simulink model "rzs10thnew2021b"  (R2021b)
settings: Solver=FixedStepDiscrete  StartTime=0.0  StopTime=10.0  FixedStep=0.001  RelTol=1e-3  EnableMultiTasking=on
values from neighbouring files (symbols this model uses):
  F = 0.0    [rzdatabase.sldd]
  T = 1.0    [rzdatabase.sldd]
libraries: simulink x143, hdlsllib x95, spsEdgeDetectorLib x3
(part 2 of 3)

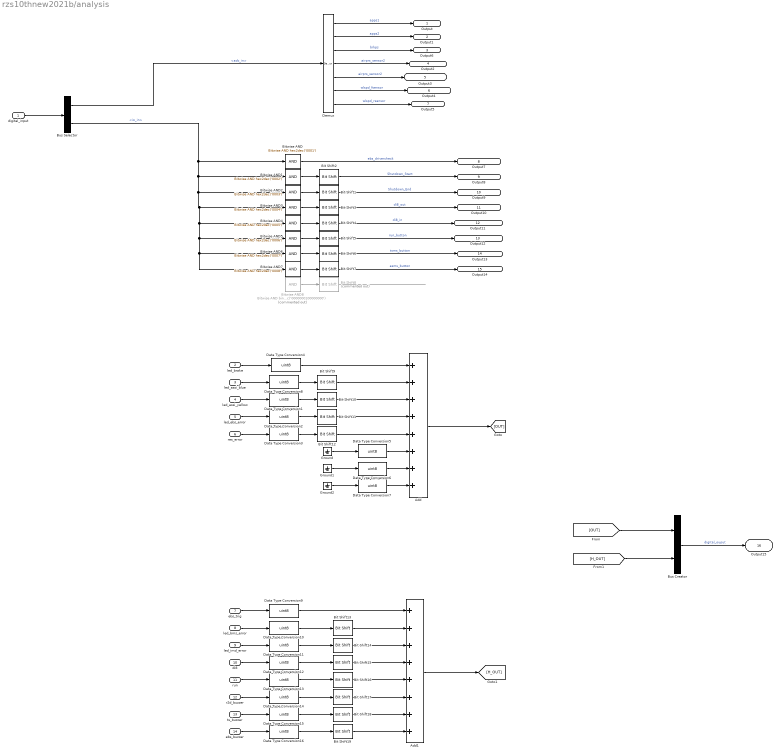
== system rzs10thnew2021b/analysis ==
  digital_input : Inport
  led_brake : Inport  Port=2
  led_assi_blue : Inport  Port=3
  led_assi_yellow : Inport  Port=4
  led_ebs_error : Inport  Port=5
  res_error : Inport  Port=6
  ebs_trig : Inport  Port=7
  led_bms_error : Inport  Port=8
  led_imd_error : Inport  Port=9
  di8 : Inport  Port=10
  run : Inport  Port=11
  r2d_buzzer : Inport  Port=12
  ts_buzzer : Inport  Port=13
  ebs_buzzer : Inport  Port=14
  Add : Sum  Inputs=++++++++
  Add1 : Sum  Inputs=++++++++
  Bit Shift1 : hdlsllib/Logic and Bit Operations/Bit Shift  mode=Shift Right Logical  N=2
  Bit Shift10 : hdlsllib/Logic and Bit Operations/Bit Shift  mode=Shift Right Logical  N=2
  Bit Shift11 : hdlsllib/Logic and Bit Operations/Bit Shift  mode=Shift Right Logical  N=3
  Bit Shift12 : hdlsllib/Logic and Bit Operations/Bit Shift  mode=Shift Right Logical  N=4
  Bit Shift13 : hdlsllib/Logic and Bit Operations/Bit Shift  mode=Shift Left Logical  N=1
  Bit Shift14 : hdlsllib/Logic and Bit Operations/Bit Shift  mode=Shift Left Logical  N=2
  Bit Shift15 : hdlsllib/Logic and Bit Operations/Bit Shift  mode=Shift Left Logical  N=3
  Bit Shift16 : hdlsllib/Logic and Bit Operations/Bit Shift  mode=Shift Left Logical  N=4
  Bit Shift17 : hdlsllib/Logic and Bit Operations/Bit Shift  mode=Shift Left Logical  N=5
  Bit Shift18 : hdlsllib/Logic and Bit Operations/Bit Shift  mode=Shift Left Logical  N=6
  Bit Shift19 : hdlsllib/Logic and Bit Operations/Bit Shift  mode=Shift Left Logical  N=7
  Bit Shift2 : hdlsllib/Logic and Bit Operations/Bit Shift  mode=Shift Right Logical  N=1
  Bit Shift3 : hdlsllib/Logic and Bit Operations/Bit Shift  mode=Shift Right Logical  N=3
  Bit Shift4 : hdlsllib/Logic and Bit Operations/Bit Shift  mode=Shift Right Logical  N=4
  Bit Shift5 : hdlsllib/Logic and Bit Operations/Bit Shift  mode=Shift Right Logical  N=5
  Bit Shift6 : hdlsllib/Logic and Bit Operations/Bit Shift  mode=Shift Right Logical  N=6
  Bit Shift7 : hdlsllib/Logic and Bit Operations/Bit Shift  mode=Shift Right Logical  N=7
  Bit Shift8 : hdlsllib/Logic and Bit Operations/Bit Shift  Commented=on  mode=Shift Right Logical  N=8
  Bit Shift9 : hdlsllib/Logic and Bit Operations/Bit Shift  mode=Shift Left Logical  N=1
  Bitwise AND : simulink/Logic and Bit Operations/Bitwise Operator  logicop=AND  UseBitMask=on  BitMask=hex2dec('0001')  BitMaskRealWorld=Stored Integer
  Bitwise AND1 : simulink/Logic and Bit Operations/Bitwise Operator  logicop=AND  UseBitMask=on  BitMask=hex2dec('0002')  BitMaskRealWorld=Stored Integer
  Bitwise AND2 : simulink/Logic and Bit Operations/Bitwise Operator  logicop=AND  UseBitMask=on  BitMask=hex2dec('0003')  BitMaskRealWorld=Stored Integer
  Bitwise AND3 : simulink/Logic and Bit Operations/Bitwise Operator  logicop=AND  UseBitMask=on  BitMask=hex2dec('0004')  BitMaskRealWorld=Stored Integer
  Bitwise AND4 : simulink/Logic and Bit Operations/Bitwise Operator  logicop=AND  UseBitMask=on  BitMask=hex2dec('0005')  BitMaskRealWorld=Stored Integer
  Bitwise AND5 : simulink/Logic and Bit Operations/Bitwise Operator  logicop=AND  UseBitMask=on  BitMask=hex2dec('0006')  BitMaskRealWorld=Stored Integer
  Bitwise AND6 : simulink/Logic and Bit Operations/Bitwise Operator  logicop=AND  UseBitMask=on  BitMask=hex2dec('0007')  BitMaskRealWorld=Stored Integer
  Bitwise AND7 : simulink/Logic and Bit Operations/Bitwise Operator  logicop=AND  UseBitMask=on  BitMask=hex2dec('0008')  BitMaskRealWorld=Stored Integer
  Bitwise AND8 : simulink/Logic and Bit Operations/Bitwise Operator  Commented=on  logicop=AND  UseBitMask=on  BitMask=bin2dec('0000000100000000')  BitMaskRealWorld=Stored Integer
  Bus Creator : BusCreator  Inputs=2  OutDataTypeStr=Bus: VCU_OUT_PAR  NonVirtualBus=on
      settings: InheritFromInputs=off
  Bus Selector : BusSelector  OutputSignals=adc_in,io_in
  Data Type Conversion{1..16} (16 alike) : DataTypeConversion  OutDataTypeStr=uint8
  Demux : Demux  Outputs=7
  Ground : Ground
  Ground1 : Ground
  Ground2 : Ground
  Output : Outport
  Output1 : Outport  Port=2
  Output6 : Outport  Port=3
  Output2 : Outport  Port=4
  Output3 : Outport  Port=5
  Output4 : Outport  Port=6
  Output5 : Outport  Port=7
  Output7 : Outport  Port=8
  Output8 : Outport  Port=9
  Output9 : Outport  Port=10
  Output10 : Outport  Port=11
  Output11 : Outport  Port=12
  Output12 : Outport  Port=13
  Output13 : Outport  Port=14
  Output14 : Outport  Port=15
  Output15 : Outport  Port=16
  wires:
  Bitwise AND1/1 -> Bit Shift2/1
  Bitwise AND2/1 -> Bit Shift1/1
  Bitwise AND3/1 -> Bit Shift3/1
  Bitwise AND4/1 -> Bit Shift4/1
  Bitwise AND5/1 -> Bit Shift5/1
  Bitwise AND6/1 -> Bit Shift6/1
  Bitwise AND7/1 -> Bit Shift7/1
  Bitwise AND8/1 -> Bit Shift8/1
  Bit Shift2/1 -> Output8/1  "Shutdown_Start"
  Bit Shift1/1 -> Output9/1  "Shutdown_End"
  Bit Shift3/1 -> Output10/1  "di8_out"
  Bit Shift4/1 -> Output11/1  "di8_in"
  Bit Shift5/1 -> Output12/1  "run_button"
  Bit Shift6/1 -> Output13/1  "tsms_button"
  Bit Shift7/1 -> Output14/1  "asms_button"
  Bit Shift8/1 -> ?
  Bitwise AND/1 -> Output7/1  "ebs_drivercheck"
  Ground2/1 -> Data Type Conversion7/1
  Ground1/1 -> Data Type Conversion6/1
  Ground/1 -> Data Type Conversion5/1
  Bit Shift13/1 -> Add1/2
  Bit Shift14/1 -> Add1/3
  Bit Shift15/1 -> Add1/4
  Bit Shift16/1 -> Add1/5
  Bit Shift17/1 -> Add1/6
  Bit Shift18/1 -> Add1/7
  Bit Shift19/1 -> Add1/8
  led_brake/1 -> Data Type Conversion4/1
  Data Type Conversion4/1 -> Add/1
  Bit Shift9/1 -> Add/2
  Bit Shift10/1 -> Add/3
  Bit Shift11/1 -> Add/4
  Bit Shift12/1 -> Add/5
  Data Type Conversion5/1 -> Add/6
  Data Type Conversion6/1 -> Add/7
  Data Type Conversion7/1 -> Add/8
  led_assi_blue/1 -> Data Type Conversion8/1
  Data Type Conversion8/1 -> Bit Shift9/1
  led_assi_yellow/1 -> Data Type Conversion1/1
  Data Type Conversion1/1 -> Bit Shift10/1
  led_ebs_error/1 -> Data Type Conversion2/1
  Data Type Conversion2/1 -> Bit Shift11/1
  res_error/1 -> Data Type Conversion3/1
  Data Type Conversion3/1 -> Bit Shift12/1
  ebs_trig/1 -> Data Type Conversion9/1
  Data Type Conversion9/1 -> Add1/1
  led_bms_error/1 -> Data Type Conversion10/1
  Data Type Conversion10/1 -> Bit Shift13/1
  led_imd_error/1 -> Data Type Conversion11/1
  Data Type Conversion11/1 -> Bit Shift14/1
  di8/1 -> Data Type Conversion12/1
  Data Type Conversion12/1 -> Bit Shift15/1
  run/1 -> Data Type Conversion13/1
  Data Type Conversion13/1 -> Bit Shift16/1
  r2d_buzzer/1 -> Data Type Conversion14/1
  Data Type Conversion14/1 -> Bit Shift17/1
  ts_buzzer/1 -> Data Type Conversion15/1
  Data Type Conversion15/1 -> Bit Shift18/1
  ebs_buzzer/1 -> Data Type Conversion16/1
  Data Type Conversion16/1 -> Bit Shift19/1
  Demux/1 -> Output/1  "apps1"
  Demux/2 -> Output1/1  "apps2"
  Demux/3 -> Output6/1  "brkps"
  Demux/5 -> Output3/1  "airprs_sensor2"
  Demux/6 -> Output4/1  "wlspd_fsensor"
  Demux/7 -> Output5/1  "wlspd_rsensor"
  Bus Creator/1 -> Output15/1  "digital_ouput"
  Demux/4 -> Output2/1  "airprs_sensor2"
  Add1/1 -> [H_OUT]
  Add/1 -> [OUT]
  [H_OUT] -> Bus Creator/2
  [OUT] -> Bus Creator/1
  Bus Selector/1 -> Demux/1  "<adc_in>"
  Bus Selector/2 -> Bitwise AND7/1, Bitwise AND6/1, Bitwise AND5/1, Bitwise AND4/1, Bitwise AND3/1, Bitwise AND2/1, Bitwise AND1/1, Bitwise AND/1  "<io_in>"
  digital_input/1 -> Bus Selector/1

== system rzs10thnew2021b/AMI_CAN/AMI_Receivemsg ==
  AMI_Tx : Inport
  Bit Shift : hdlsllib/Logic and Bit Operations/Bit Shift  mode=Shift Right Logical  N=4
  Bitwise AND : simulink/Logic and Bit Operations/Bitwise Operator  logicop=AND  UseBitMask=on  BitMask=bin2dec('11110000')  BitMaskRealWorld=Stored Integer
  Demux : Demux  Outputs=8
  Mux : Mux  Inputs=8
  ami_astask : Outport
  Output : Outport  Port=2
  wires:
  Demux/6 -> Mux/6
  Demux/2 -> Mux/2
  Demux/4 -> Mux/4
  AMI_Tx/1 -> Demux/1
  Demux/7 -> Mux/7
  Demux/5 -> Mux/5
  Demux/8 -> Mux/8
  Demux/3 -> Mux/3
  Demux/1 -> Mux/1, Bitwise AND/1
  Bitwise AND/1 -> Bit Shift/1
  Bit Shift/1 -> ami_astask/1
  Mux/1 -> Output/1

== system rzs10thnew2021b/AMI_CAN/AMI_Transmitmsg ==
  as_flag_state : Inport
  task_finish : Inport  Port=2
  Add1 : Sum
  Bit Shift : hdlsllib/Logic and Bit Operations/Bit Shift  mode=Shift Left Logical  N=1
  Bitwise AND : simulink/Logic and Bit Operations/Bitwise Operator  logicop=AND  UseBitMask=on  BitMask=bin2dec('01111111')  BitMaskRealWorld=Stored Integer
  Bus Selector : BusSelector  OutputSignals=as_off_flag,manual_driving_flag,as_ready_flag,r2d_flag,as_driving_flag,as_finished_flag,as_emergency_flag
  Chart : Stateflow chart  TreatAsAtomicUnit=on
  Ground{,1..6} (7 alike) : Ground
  Mux : Mux  Inputs=8
  Signal Conversion : SignalConversion  OverrideOpt=off
  Output : Outport
  wires:
  as_flag_state/1 -> Bus Selector/1
  Bitwise AND/1 -> Bit Shift/1
  Bit Shift/1 -> Add1/1
  task_finish/1 -> Add1/2
  Add1/1 -> Mux/1
  Bus Selector/1 -> Chart/1(as_off_flag)  "<as_off_flag>"
  Bus Selector/2 -> Chart/2(munual_driving_flag)  "<manual_driving_flag>"
  Bus Selector/3 -> Chart/3(as_ready_flag)  "<as_ready_flag>"
  Bus Selector/4 -> Chart/4(r2d_flag)  "<r2d_flag>"
  Bus Selector/5 -> Chart/5(as_driving_flag)  "<as_driving_flag>"
  Bus Selector/6 -> Chart/6(as_finished_flag)  "<as_finished_flag>"
  Bus Selector/7 -> Chart/7(as_emergency_flag)  "<as_emergency_flag>"
  Chart/1(ami_process) -> Bitwise AND/1
  Ground/1 -> Mux/2
  Ground1/1 -> Mux/3
  Ground2/1 -> Mux/4
  Ground3/1 -> Mux/5
  Ground4/1 -> Mux/6
  Ground5/1 -> Mux/7
  Ground6/1 -> Mux/8
  Mux/1 -> Signal Conversion/1
  Signal Conversion/1 -> Output/1

== system rzs10thnew2021b/ASB_Selfcheck/Brake_Sensor_Check ==
  note: 下四路为有效制动阈值油压
  note: 上四路油压信号阈值为非制动状态油压
  note: 所有常数待定
  airprs_sensor1 : Inport
  oilprs_frsensor : Inport  Port=2
  oilprs_rrsensor : Inport  Port=3
  oilprs_flsensor : Inport  Port=4
  oilprs_rlsensor : Inport  Port=5
  Compare To Constant : simulink/Logic and Bit Operations/Compare To Constant  relop=>=  const=0.74  OutDataTypeStr=boolean
  Compare To Constant{1,3,5,7} (4 alike) : simulink/Logic and Bit Operations/Compare To Constant  relop=>=  const=0.848  OutDataTypeStr=boolean
  Compare To Constant{2,4,6,8} (4 alike) : simulink/Logic and Bit Operations/Compare To Constant  relop=>=  const=0.742  OutDataTypeStr=boolean
  Logical Operator : Logic  Inputs=5  AllPortsSameDT=off  OutDataTypeStr=boolean
  Logical Operator1 : Logic  Inputs=4  AllPortsSameDT=off  OutDataTypeStr=boolean
  brksensor_check : Outport
  brake_on : Outport  Port=2
  wires:
  airprs_sensor1/1 -> Compare To Constant/1
  oilprs_frsensor/1 -> Compare To Constant5/1, Compare To Constant1/1
  oilprs_rrsensor/1 -> Compare To Constant7/1, Compare To Constant3/1
  oilprs_flsensor/1 -> Compare To Constant6/1, Compare To Constant2/1
  oilprs_rlsensor/1 -> Compare To Constant8/1, Compare To Constant4/1
  Compare To Constant3/1 -> Logical Operator/3
  Compare To Constant/1 -> Logical Operator/1
  Compare To Constant1/1 -> Logical Operator/2
  Compare To Constant2/1 -> Logical Operator/4
  Compare To Constant4/1 -> Logical Operator/5
  Logical Operator/1 -> brksensor_check/1
  Logical Operator1/1 -> brake_on/1
  Compare To Constant5/1 -> Logical Operator1/1
  Compare To Constant7/1 -> Logical Operator1/2
  Compare To Constant6/1 -> Logical Operator1/3
  Compare To Constant8/1 -> Logical Operator1/4

== system rzs10thnew2021b/ASB_Selfcheck/EBS_On_Check ==
  airprs_sensor2 : Inport
  Compare To Constant : simulink/Logic and Bit Operations/Compare To Constant  relop=>=  const=0.9  OutDataTypeStr=boolean
  ebs_working : Outport
  wires:
  airprs_sensor2/1 -> Compare To Constant/1
  Compare To Constant/1 -> ebs_working/1

== system rzs10thnew2021b/AS_Stateflow/Car_Spdzero_Check ==
  wlspd_fsensor : Inport
  wlspd_hsensor : Inport  Port=2
  Compare To Constant : simulink/Logic and Bit Operations/Compare To Constant  relop===  const=0  OutDataTypeStr=boolean
  Compare To Constant1 : simulink/Logic and Bit Operations/Compare To Constant  relop===  const=0  OutDataTypeStr=boolean
  Dead Zone : DeadZone  SaturateOnIntegerOverflow=on
  Dead Zone1 : DeadZone  SaturateOnIntegerOverflow=on
  Logical Operator : Logic  AllPortsSameDT=off  OutDataTypeStr=boolean
  car_spdzero : Outport
  wires:
  wlspd_fsensor/1 -> Dead Zone/1
  wlspd_hsensor/1 -> Dead Zone1/1
  Dead Zone/1 -> Compare To Constant/1
  Dead Zone1/1 -> Compare To Constant1/1
  Compare To Constant/1 -> Logical Operator/1
  Compare To Constant1/1 -> Logical Operator/2
  Logical Operator/1 -> car_spdzero/1

== system rzs10thnew2021b/EPS/EPS_ReceiveMsg ==
  canb_epssendmsg1 : Inport
  canb_epssendmsg2 : Inport  Port=2
  EPS_Send_Msg1 : Subsystem
  EPS_Send_Msg2 : Subsystem
  canb_epssendmsg1signal : Outport
  canb_epssendmsg2signal : Outport  Port=2
  wires:
  canb_epssendmsg1/1 -> EPS_Send_Msg1/1(canb_epssendmsg1)
  EPS_Send_Msg1/1(canb_epssendmsg1signal) -> canb_epssendmsg1signal/1
  canb_epssendmsg2/1 -> EPS_Send_Msg2/1(canb_epssendmsg2)
  EPS_Send_Msg2/1(canb_epssendmsg2signal) -> canb_epssendmsg2signal/1

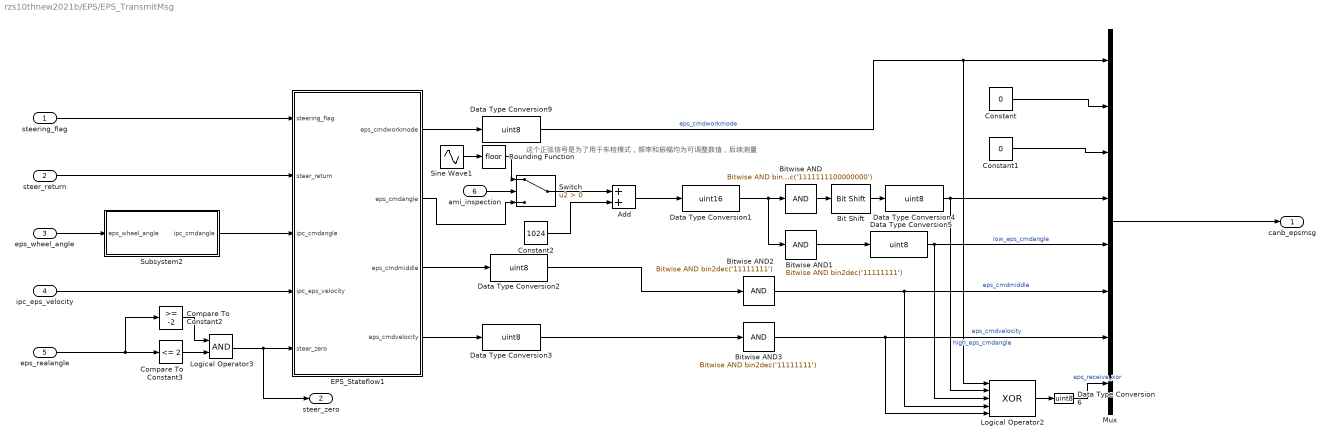
== system rzs10thnew2021b/EPS/EPS_TransmitMsg ==
  note: 这个正弦信号是为了用于车检模式，频率和振幅均为可调整数值，后续测量
  steering_flag : Inport
  steer_return : Inport  Port=2
  eps_wheel_angle : Inport  Port=3
  ipc_eps_velocity : Inport  Port=4
  eps_realangle : Inport  Port=5
  ami_inspection : Inport  Port=6
  Add : Sum
  Bit Shift : hdlsllib/Logic and Bit Operations/Bit Shift  mode=Shift Right Logical  N=8
  Bitwise AND : simulink/Logic and Bit Operations/Bitwise Operator  logicop=AND  UseBitMask=on  BitMask=bin2dec('1111111100000000')  BitMaskRealWorld=Stored Integer
  Bitwise AND1 : simulink/Logic and Bit Operations/Bitwise Operator  logicop=AND  UseBitMask=on  BitMask=bin2dec('11111111')  BitMaskRealWorld=Stored Integer
  Bitwise AND2 : simulink/Logic and Bit Operations/Bitwise Operator  logicop=AND  UseBitMask=on  BitMask=bin2dec('11111111')  BitMaskRealWorld=Stored Integer
  Bitwise AND3 : simulink/Logic and Bit Operations/Bitwise Operator  logicop=AND  UseBitMask=on  BitMask=bin2dec('11111111')  BitMaskRealWorld=Stored Integer
  Compare To Constant2 : simulink/Logic and Bit Operations/Compare To Constant  relop=>=  const=-2  OutDataTypeStr=boolean
  Compare To Constant3 : simulink/Logic and Bit Operations/Compare To Constant  relop=<=  const=2  OutDataTypeStr=boolean
  Constant : Constant  Value=0  OutDataTypeStr=uint8
  Constant1 : Constant  Value=0  OutDataTypeStr=uint8
  Constant2 : Constant  Value=1024  OutDataTypeStr=double
  Data Type Conversion1 : DataTypeConversion  OutDataTypeStr=uint16
  Data Type Conversion{2..6,9} (6 alike) : DataTypeConversion  OutDataTypeStr=uint8
  EPS_Stateflow1 : Stateflow chart  TreatAsAtomicUnit=on
  Logical Operator2 : Logic  Operator=XOR  Inputs=5  AllPortsSameDT=off  OutDataTypeStr=boolean
  Logical Operator3 : Logic  AllPortsSameDT=off  OutDataTypeStr=boolean
  Mux : Mux  Inputs=8
  Rounding Function : Rounding
  Sine Wave1 : Sin  Amplitude=90
  Subsystem2 : Subsystem
  Switch : Switch  Criteria=u2 > Threshold
  canb_epsmsg : Outport
  steer_zero : Outport  Port=2
  wires:
  Data Type Conversion5/1 -> Logical Operator2/3, Mux/5  "low_eps_cmdangle"
  Data Type Conversion9/1 -> Logical Operator2/1, Mux/1  "eps_cmdworkmode"
  Bitwise AND3/1 -> Logical Operator2/5, Mux/7  "eps_cmdvelocity"
  Compare To Constant3/1 -> Logical Operator3/2
  Data Type Conversion3/1 -> Bitwise AND3/1
  Bit Shift/1 -> Data Type Conversion4/1
  eps_realangle/1 -> Compare To Constant2/1, Compare To Constant3/1
  Data Type Conversion1/1 -> Bitwise AND/1, Bitwise AND1/1
  EPS_Stateflow1/4(eps_cmdvelocity) -> Data Type Conversion3/1
  Logical Operator3/1 -> steer_zero/1, EPS_Stateflow1/5(steer_zero)
  Bitwise AND2/1 -> Logical Operator2/4, Mux/6  "eps_cmdmiddle"
  EPS_Stateflow1/3(eps_cmdmiddle) -> Data Type Conversion2/1
  Constant1/1 -> Mux/3
  Bitwise AND/1 -> Bit Shift/1
  Data Type Conversion4/1 -> Mux/4, Logical Operator2/2  "high_eps_cmdangle"
  eps_wheel_angle/1 -> Subsystem2/1(eps_wheel_angle)
  Data Type Conversion2/1 -> Bitwise AND2/1
  Compare To Constant2/1 -> Logical Operator3/1
  Logical Operator2/1 -> Data Type Conversion6/1
  steer_return/1 -> EPS_Stateflow1/2(steer_return)
  EPS_Stateflow1/1(eps_cmdworkmode) -> Data Type Conversion9/1
  Bitwise AND1/1 -> Data Type Conversion5/1
  ipc_eps_velocity/1 -> EPS_Stateflow1/4(ipc_eps_velocity)
  Constant/1 -> Mux/2
  Subsystem2/1(ipc_cmdangle) -> EPS_Stateflow1/3(ipc_cmdangle)
  Mux/1 -> canb_epsmsg/1
  steering_flag/1 -> EPS_Stateflow1/1(steering_flag)
  Add/1 -> Data Type Conversion1/1
  Constant2/1 -> Add/2
  Data Type Conversion6/1 -> Mux/8  "eps_receive_xor"
  ami_inspection/1 -> Switch/2
  Switch/1 -> Add/1
  EPS_Stateflow1/2(eps_cmdangle) -> Switch/3
  Rounding Function/1 -> Switch/1
  Sine Wave1/1 -> Rounding Function/1

== system rzs10thnew2021b/ESP/ESP_ReceiveMsg ==
  canb_esp_t01 : Inport
  canb_esp_t03 : Inport  Port=2
  canb_esp_t06 : Inport  Port=3
  canb_esp_t07 : Inport  Port=4
  Bus Selector : BusSelector  OutputSignals=lifeSig
  ESP_T_01 : Subsystem
  ESP_T_03 : Subsystem
  ESP_T_06 : Subsystem
  ESP_T_07 : Subsystem
  Subsystem : Subsystem
  ESP_T_01sigal : Outport
  ESP_T_03signal : Outport  Port=2
  ESP_T_06signal : Outport  Port=3
  ESP_T_07signal : Outport  Port=4
  brkmotor_check : Outport  Port=5
  wires:
  canb_esp_t01/1 -> ESP_T_01/1(canb_esp_t01)
  ESP_T_01/1(ESP_T_01sigal) -> ESP_T_01sigal/1
  canb_esp_t03/1 -> ESP_T_03/1(canb_esp_t03)
  canb_esp_t06/1 -> ESP_T_06/1(canb_esp_t06)
  ESP_T_06/1(ESP_T_06signal) -> ESP_T_06signal/1
  canb_esp_t07/1 -> ESP_T_07/1(canb_esp_t07)
  ESP_T_07/1(ESP_T_07signal) -> ESP_T_07signal/1
  Subsystem/1(brkmotor_check) -> brkmotor_check/1
  ESP_T_03/1(ESP_T_03signal) -> Bus Selector/1, ESP_T_03signal/1
  Bus Selector/1 -> Subsystem/1(lifesig)  "<lifeSig>"

== system rzs10thnew2021b/ESP/ESP_TransmitMsg ==
  ipc_esp_pressure : Inport
  brake_flag : Inport  Port=2
  lifeSig : Inport  Port=3
  checkSum : Inport  Port=4
  ESP_R_00 : Subsystem
  canb_esp_r00 : Outport
  wires:
  ipc_esp_pressure/1 -> ESP_R_00/1(ipc_esp_pressure)
  brake_flag/1 -> ESP_R_00/2(brake_flag)
  ESP_R_00/1(canb_esp_r00) -> canb_esp_r00/1
  checkSum/1 -> ESP_R_00/4(checkSum)
  lifeSig/1 -> ESP_R_00/3(lifeSig)

== system rzs10thnew2021b/IPC/IPC_ReceiveMsg ==
  ipc_resgo : Inport
  ipc_resstop : Inport  Port=2
  ipc_astask : Inport  Port=3
  IPC_Rx_Msg : Subsystem
  canb_ipcrxmsg : Outport
  wires:
  ipc_resgo/1 -> IPC_Rx_Msg/1(ipc_resgo)
  ipc_resstop/1 -> IPC_Rx_Msg/2(ipc_resstop)
  ipc_astask/1 -> IPC_Rx_Msg/3(ipc_astask)
  IPC_Rx_Msg/1(canb_ipcrxmsg) -> canb_ipcrxmsg/1

== system rzs10thnew2021b/IPC/IPC_TransmitMsg ==
  canb_ipctsmsg1 : Inport
  canb_ipctsmsg2 : Inport  Port=2
  IPC_Tx_Msg1 : Subsystem
  IPC_Tx_Msg2 : Subsystem
  ipc_esp_pressure : Outport
  ipc_motor_torque : Outport  Port=2
  ipc_eps_angle : Outport  Port=3
  ipc_eps_velocity : Outport  Port=4
  ipc_err : Outport  Port=5
  task_finish : Outport  Port=6
  wires:
  canb_ipctsmsg1/1 -> IPC_Tx_Msg1/1(canb_ipctsmsg1)
  IPC_Tx_Msg1/1(ipc_esp_pressure) -> ipc_esp_pressure/1
  IPC_Tx_Msg1/2(ipc_motor_torque) -> ipc_motor_torque/1
  canb_ipctsmsg2/1 -> IPC_Tx_Msg2/1(canb_ipctsmsg2)
  IPC_Tx_Msg2/2(ipc_eps_velocity) -> ipc_eps_velocity/1
  IPC_Tx_Msg2/1(ipc_eps_angle) -> ipc_eps_angle/1
  IPC_Tx_Msg2/3(ipc_err) -> ipc_err/1
  IPC_Tx_Msg2/4(task_finish) -> task_finish/1

== system rzs10thnew2021b/LED_Control/BMS_LED ==
  bms_error : Inport
  imd_error : Inport  Port=2
  BMS_LED : Stateflow chart  TreatAsAtomicUnit=on
  IMD_LED : Stateflow chart  TreatAsAtomicUnit=on
  led_bms_error : Outport
  led_imd_error : Outport  Port=2
  wires:
  bms_error/1 -> BMS_LED/1(bms_error)
  imd_error/1 -> IMD_LED/1(imd_error)
  BMS_LED/1(led_bms_error) -> led_bms_error/1  "led_bms_error"
  IMD_LED/1(led_imd_error) -> led_imd_error/1  "led_imd_error"

== system rzs10thnew2021b/LED_Control/EBS_LED ==
  note: 液压元件失效
  note: 手动阀未关
  note: 前气路故障
  note: 上电亮灯
  note: 气动元件检测与气压检测
  note: 油压检测
  res_stop : Inport
  res_communication : Inport  Port=2
  Shutdown_Start : Inport  Port=3
  Shutdown_End : Inport  Port=4
  sensor_signal : Inport  Port=5
  ESP_T_03signal : Inport  Port=6
  asms_button : Inport  Port=7
  Bus Selector : BusSelector  OutputSignals=airprs_sensor1,airprs_sensor2
  Bus Selector1 : BusSelector  OutputSignals=oilprs_flsensor,oilprs_frsensor,oilprs_rlsensor,oilprs_rrsensor
  Compare To Constant{,3..6} (5 alike) : simulink/Logic and Bit Operations/Compare To Constant  relop=<=  const=0.11  OutDataTypeStr=boolean
  Compare To Constant1 : simulink/Logic and Bit Operations/Compare To Constant  relop=<=  const=0.5  OutDataTypeStr=boolean
  Compare To Constant2 : simulink/Logic and Bit Operations/Compare To Constant  relop=>=  const=0.78  OutDataTypeStr=boolean
  Enabled Subsystem : Subsystem  TreatAsAtomicUnit=on
  Logical Operator : Logic  Operator=OR  Inputs=5  AllPortsSameDT=off  OutDataTypeStr=boolean
  Logical Operator2 : Logic  Inputs=4  AllPortsSameDT=off  OutDataTypeStr=boolean
  Logical Operator3 : Logic  Operator=OR  Inputs=4  AllPortsSameDT=off  OutDataTypeStr=boolean
  Shutdown_Button : Stateflow chart  TreatAsAtomicUnit=on
  display : Stateflow chart  TreatAsAtomicUnit=on
  led_ebs_error : Outport
  wires:
  Compare To Constant5/1 -> Logical Operator3/3
  Bus Selector/2 -> Compare To Constant1/1, Compare To Constant2/1  "<airprs_sensor2>"
  Compare To Constant2/1 -> Enabled Subsystem/1(In1)
  Compare To Constant1/1 -> Logical Operator/2
  Logical Operator/1 -> led_ebs_error/1
  Bus Selector1/4 -> Compare To Constant6/1  "<oilprs_rrsensor>"
  Compare To Constant4/1 -> Logical Operator3/2
  Bus Selector/1 -> Compare To Constant/1  "<airprs_sensor1>"
  Compare To Constant6/1 -> Logical Operator3/4
  Bus Selector1/1 -> Compare To Constant3/1  "<oilprs_flsensor>"
  display/1(spark) -> Logical Operator/5
  Logical Operator3/1 -> Logical Operator/4
  asms_button/1 -> Logical Operator2/4
  Logical Operator2/1 -> Enabled Subsystem/Enable
  Compare To Constant/1 -> Logical Operator/1
  Enabled Subsystem/1(Out1) -> Logical Operator/3
  Shutdown_Button/1(shutdown_flag) -> Logical Operator2/3
  Compare To Constant3/1 -> Logical Operator3/1
  Bus Selector1/2 -> Compare To Constant4/1  "<oilprs_frsensor>"
  Bus Selector1/3 -> Compare To Constant5/1  "<oilprs_rlsensor>"
  ESP_T_03signal/1 -> Bus Selector1/1
  res_stop/1 -> Logical Operator2/1
  res_communication/1 -> Logical Operator2/2
  Shutdown_End/1 -> Shutdown_Button/2(Shutdown_End)
  Shutdown_Start/1 -> Shutdown_Button/1(Shutdown_Start)
  sensor_signal/1 -> Bus Selector/1

== system rzs10thnew2021b/LED_Control/Subsystem ==
  as_led_blue1 : Inport
  asms_button : Inport  Port=2
  Constant : Constant  Value=0
  Constant1 : Constant  Value=0
  Constant2 : Constant
  Data Type Conversion : DataTypeConversion  OutDataTypeStr=boolean
  Pulse Generator : DiscretePulseGenerator  Period=100  PulseWidth=50  SampleTime=-1
  Switch : Switch  Criteria=u2 > Threshold  Threshold=10
  Switch1 : Switch  Criteria=u2 > Threshold  Threshold=10
  Switch2 : Switch  Criteria=u2 > Threshold  Threshold=40000
  blue : Stateflow chart  TreatAsAtomicUnit=on
  led_assi_blue : Outport
  wires:
  as_led_blue1/1 -> blue/1(as_led_blue)
  Switch2/1 -> Data Type Conversion/1
  Switch/1 -> Switch2/2
  Constant2/1 -> Switch2/1
  [blue] -> Switch1/2
  Constant1/1 -> Switch1/3
  Data Type Conversion/1 -> led_assi_blue/1
  Switch1/1 -> Switch2/3
  [blue] -> Switch/1
  Pulse Generator/1 -> Switch1/1
  blue/1(blue) -> [blue]
  [blue] -> Switch/2
  Constant/1 -> Switch/3
  asms_button/1 -> blue/2(asms_button)

== system rzs10thnew2021b/LED_Control/Subsystem1 ==
  asms_button : Inport
  as_led_yellow : Inport  Port=2
  Constant : Constant  Value=0
  Constant1 : Constant  Value=0
  Constant3 : Constant
  Data Type Conversion : DataTypeConversion  OutDataTypeStr=boolean
  Pulse Generator : DiscretePulseGenerator  Period=100  PulseWidth=50  SampleTime=-1
  Switch : Switch  Criteria=u2 > Threshold  Threshold=10
  Switch1 : Switch  Criteria=u2 > Threshold  Threshold=10
  Switch2 : Switch  Criteria=u2 > Threshold  Threshold=40000
  yellow : Stateflow chart  TreatAsAtomicUnit=on
  led_assi_yellow : Outport
  wires:
  [yellow] -> Switch/2
  Switch1/1 -> Switch2/3
  Switch2/1 -> Data Type Conversion/1
  Constant3/1 -> Switch2/1
  yellow/1(yellow) -> [yellow]
  as_led_yellow/1 -> yellow/1(as_led_yellow)
  Switch/1 -> Switch2/2
  Pulse Generator/1 -> Switch1/1
  Data Type Conversion/1 -> led_assi_yellow/1
  [yellow] -> Switch1/2
  Constant/1 -> Switch/3
  [yellow] -> Switch/1
  Constant1/1 -> Switch1/3
  asms_button/1 -> yellow/2(asms_button)

== system rzs10thnew2021b/Motor_Control/AS_Torque_Calculation ==
  ipc_motor_torque : Inport
  Enable : EnablePort
  Data Type Conversion : DataTypeConversion  OutDataTypeStr=double
  Saturation : Saturate  UpperLimit=55  LowerLimit=0
  as_torque : Outport
  wires:
  ipc_motor_torque/1 -> Saturation/1
  Saturation/1 -> Data Type Conversion/1
  Data Type Conversion/1 -> as_torque/1

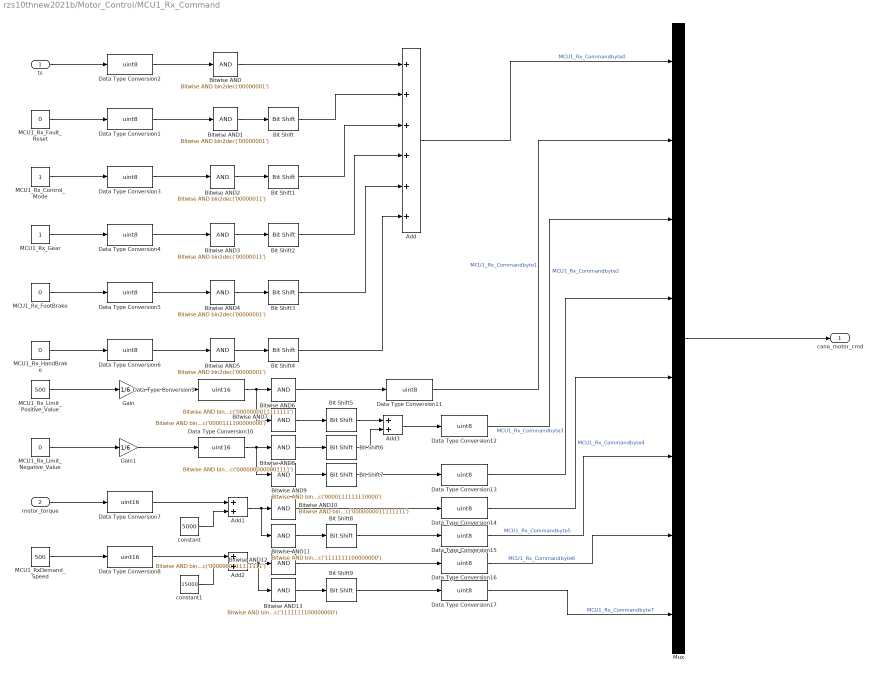
== system rzs10thnew2021b/Motor_Control/MCU1_Rx_Command ==
  ts : Inport
  motor_torque : Inport  Port=2
  Add : Sum  Inputs=++++++
  Add1 : Sum
  Add2 : Sum
  Add3 : Sum
  Bit Shift : hdlsllib/Logic and Bit Operations/Bit Shift  mode=Shift Left Logical  N=1
  Bit Shift1 : hdlsllib/Logic and Bit Operations/Bit Shift  mode=Shift Left Logical  N=2
  Bit Shift2 : hdlsllib/Logic and Bit Operations/Bit Shift  mode=Shift Left Logical  N=4
  Bit Shift3 : hdlsllib/Logic and Bit Operations/Bit Shift  mode=Shift Left Logical  N=6
  Bit Shift4 : hdlsllib/Logic and Bit Operations/Bit Shift  mode=Shift Left Logical  N=7
  Bit Shift5 : hdlsllib/Logic and Bit Operations/Bit Shift  mode=Shift Right Logical  N=8
  Bit Shift6 : hdlsllib/Logic and Bit Operations/Bit Shift  mode=Shift Left Logical  N=4
  Bit Shift7 : hdlsllib/Logic and Bit Operations/Bit Shift  mode=Shift Right Logical  N=4
  Bit Shift8 : hdlsllib/Logic and Bit Operations/Bit Shift  mode=Shift Right Logical  N=8
  Bit Shift9 : hdlsllib/Logic and Bit Operations/Bit Shift  mode=Shift Right Logical  N=8
  Bitwise AND{,1,4..5} (4 alike) : simulink/Logic and Bit Operations/Bitwise Operator  logicop=AND  UseBitMask=on  BitMask=bin2dec('00000001')  BitMaskRealWorld=Stored Integer
  Bitwise AND10 : simulink/Logic and Bit Operations/Bitwise Operator  logicop=AND  UseBitMask=on  BitMask=bin2dec('0000000011111111')  BitMaskRealWorld=Stored Integer
  Bitwise AND11 : simulink/Logic and Bit Operations/Bitwise Operator  logicop=AND  UseBitMask=on  BitMask=bin2dec('1111111100000000')  BitMaskRealWorld=Stored Integer
  Bitwise AND12 : simulink/Logic and Bit Operations/Bitwise Operator  logicop=AND  UseBitMask=on  BitMask=bin2dec('0000000011111111')  BitMaskRealWorld=Stored Integer
  Bitwise AND13 : simulink/Logic and Bit Operations/Bitwise Operator  logicop=AND  UseBitMask=on  BitMask=bin2dec('1111111100000000')  BitMaskRealWorld=Stored Integer
  Bitwise AND2 : simulink/Logic and Bit Operations/Bitwise Operator  logicop=AND  UseBitMask=on  BitMask=bin2dec('00000011')  BitMaskRealWorld=Stored Integer
  Bitwise AND3 : simulink/Logic and Bit Operations/Bitwise Operator  logicop=AND  UseBitMask=on  BitMask=bin2dec('00000011')  BitMaskRealWorld=Stored Integer
  Bitwise AND6 : simulink/Logic and Bit Operations/Bitwise Operator  logicop=AND  UseBitMask=on  BitMask=bin2dec('0000000011111111')  BitMaskRealWorld=Stored Integer
  Bitwise AND7 : simulink/Logic and Bit Operations/Bitwise Operator  logicop=AND  UseBitMask=on  BitMask=bin2dec('0000111100000000')  BitMaskRealWorld=Stored Integer
  Bitwise AND8 : simulink/Logic and Bit Operations/Bitwise Operator  logicop=AND  UseBitMask=on  BitMask=bin2dec('0000000000001111')  BitMaskRealWorld=Stored Integer
  Bitwise AND9 : simulink/Logic and Bit Operations/Bitwise Operator  logicop=AND  UseBitMask=on  BitMask=bin2dec('0000111111110000')  BitMaskRealWorld=Stored Integer
  Data Type Conversion{1..6,11..17} (13 alike) : DataTypeConversion  OutDataTypeStr=uint8
  Data Type Conversion{7..10} (4 alike) : DataTypeConversion  OutDataTypeStr=uint16
  Gain : Gain  Gain=1/6
  Gain1 : Gain  Gain=1/6
  MCU1_RxDemand_Speed : Constant  Value=500
  MCU1_Rx_Control_Mode : Constant
  MCU1_Rx_Fault_Reset : Constant  Value=0
  MCU1_Rx_FootBrake : Constant  Value=0
  MCU1_Rx_Gear : Constant
  MCU1_Rx_HandBrake : Constant  Value=0
  MCU1_Rx_Limit_Negative_Value : Constant  Value=0  OutDataTypeStr=double
  MCU1_Rx_Limit_Positive_Value : Constant  Value=500  OutDataTypeStr=double
  Mux : Mux  Inputs=8
  constant : Constant  Value=5000  OutDataTypeStr=uint16
  constant1 : Constant  Value=15000  OutDataTypeStr=uint16
  cana_motor_cmd : Outport
  wires:
  ts/1 -> Data Type Conversion2/1
  MCU1_Rx_Fault_Reset/1 -> Data Type Conversion1/1
  MCU1_Rx_Control_Mode/1 -> Data Type Conversion3/1
  MCU1_Rx_Gear/1 -> Data Type Conversion4/1
  MCU1_Rx_FootBrake/1 -> Data Type Conversion5/1
  MCU1_Rx_HandBrake/1 -> Data Type Conversion6/1
  MCU1_Rx_Limit_Positive_Value/1 -> Gain/1
  MCU1_Rx_Limit_Negative_Value/1 -> Gain1/1
  MCU1_RxDemand_Speed/1 -> Data Type Conversion8/1
  Data Type Conversion2/1 -> Bitwise AND/1
  Data Type Conversion1/1 -> Bitwise AND1/1
  Bitwise AND1/1 -> Bit Shift/1
  Data Type Conversion3/1 -> Bitwise AND2/1
  Bitwise AND2/1 -> Bit Shift1/1
  Data Type Conversion4/1 -> Bitwise AND3/1
  Bitwise AND3/1 -> Bit Shift2/1
  Data Type Conversion5/1 -> Bitwise AND4/1
  Bitwise AND4/1 -> Bit Shift3/1
  Data Type Conversion6/1 -> Bitwise AND5/1
  Bitwise AND5/1 -> Bit Shift4/1
  Bitwise AND/1 -> Add/1
  Bit Shift/1 -> Add/2
  Bit Shift1/1 -> Add/3
  Bit Shift2/1 -> Add/4
  Bit Shift3/1 -> Add/5
  Bit Shift4/1 -> Add/6
  Add/1 -> Mux/1  "MCU1_Rx_Commandbyte0"
  motor_torque/1 -> Data Type Conversion7/1
  Data Type Conversion7/1 -> Add1/1
  constant/1 -> Add1/2
  Data Type Conversion8/1 -> Add2/1
  constant1/1 -> Add2/2
  Gain/1 -> Data Type Conversion9/1
  Data Type Conversion9/1 -> Bitwise AND7/1, Bitwise AND6/1
  Bitwise AND6/1 -> Data Type Conversion11/1
  Bitwise AND7/1 -> Bit Shift5/1
  Gain1/1 -> Data Type Conversion10/1
  Data Type Conversion10/1 -> Bitwise AND9/1, Bitwise AND8/1
  Data Type Conversion11/1 -> Mux/2  "MCU1_Rx_Commandbyte1"
  Bit Shift5/1 -> Add3/1
  Bitwise AND8/1 -> Bit Shift6/1
  Bit Shift6/1 -> Add3/2
  Add3/1 -> Data Type Conversion12/1
  Data Type Conversion12/1 -> Mux/3  "MCU1_Rx_Commandbyte2"
  Bitwise AND9/1 -> Bit Shift7/1
  Bit Shift7/1 -> Data Type Conversion13/1
  Data Type Conversion13/1 -> Mux/4  "MCU1_Rx_Commandbyte3"
  Add1/1 -> Bitwise AND11/1, Bitwise AND10/1
  Bitwise AND10/1 -> Data Type Conversion14/1
  Data Type Conversion14/1 -> Mux/5  "MCU1_Rx_Commandbyte4"
  Bitwise AND11/1 -> Bit Shift8/1
  Bit Shift8/1 -> Data Type Conversion15/1
  Data Type Conversion15/1 -> Mux/6  "MCU1_Rx_Commandbyte5"
  Bit Shift9/1 -> Data Type Conversion17/1
  Bitwise AND13/1 -> Bit Shift9/1
  Bitwise AND12/1 -> Data Type Conversion16/1
  Add2/1 -> Bitwise AND13/1, Bitwise AND12/1
  Data Type Conversion16/1 -> Mux/7  "MCU1_Rx_Commandbyte6"
  Data Type Conversion17/1 -> Mux/8  "MCU1_Rx_Commandbyte7"
  Mux/1 -> cana_motor_cmd/1

== system rzs10thnew2021b/Motor_Control/MCU1_Rx_Command3 ==
  Bit Shift : hdlsllib/Logic and Bit Operations/Bit Shift  mode=Shift Right Logical  N=8
  Bit Shift1 : hdlsllib/Logic and Bit Operations/Bit Shift  mode=Shift Right Logical  N=8
  Bitwise AND : simulink/Logic and Bit Operations/Bitwise Operator  logicop=AND  UseBitMask=on  BitMask=bin2dec('0000000011111111')  BitMaskRealWorld=Stored Integer
  Bitwise AND1 : simulink/Logic and Bit Operations/Bitwise Operator  logicop=AND  UseBitMask=on  BitMask=bin2dec('1111111100000000')  BitMaskRealWorld=Stored Integer
  Bitwise AND2 : simulink/Logic and Bit Operations/Bitwise Operator  logicop=AND  UseBitMask=on  BitMask=bin2dec('0000000011111111')  BitMaskRealWorld=Stored Integer
  Bitwise AND3 : simulink/Logic and Bit Operations/Bitwise Operator  logicop=AND  UseBitMask=on  BitMask=bin2dec('1111111100000000')  BitMaskRealWorld=Stored Integer
  Data Type Conversion1 : DataTypeConversion  OutDataTypeStr=uint16
  Data Type Conversion{2..4,6} (4 alike) : DataTypeConversion  OutDataTypeStr=uint8
  Data Type Conversion5 : DataTypeConversion  OutDataTypeStr=uint16
  Mux : Mux  Inputs=8
  constant : Constant  Value=0  OutDataTypeStr=uint8
  f32__speed_KI : Constant  Value=9.3
  f32__speed_KP : Constant  Value=93
  cana_motor_cmd3 : Outport
  wires:
  f32__speed_KP/1 -> Data Type Conversion5/1
  f32__speed_KI/1 -> Data Type Conversion1/1
  Data Type Conversion5/1 -> Bitwise AND1/1, Bitwise AND/1
  Bitwise AND/1 -> Data Type Conversion2/1
  Data Type Conversion2/1 -> Mux/1  "MCU1_Rx_Command3byte0"
  Bit Shift/1 -> Data Type Conversion3/1
  Bitwise AND1/1 -> Bit Shift/1
  Data Type Conversion3/1 -> Mux/2  "MCU1_Rx_Command3byte1"
  Bitwise AND2/1 -> Data Type Conversion4/1
  Bit Shift1/1 -> Data Type Conversion6/1
  Data Type Conversion6/1 -> Mux/4  "MCU1_Rx_Command3byte3"
  Data Type Conversion1/1 -> Bitwise AND3/1, Bitwise AND2/1
  Data Type Conversion4/1 -> Mux/3  "MCU1_Rx_Command3byte2"
  Bitwise AND3/1 -> Bit Shift1/1
  constant/1 -> Mux/8, Mux/7, Mux/6, Mux/5
  Mux/1 -> cana_motor_cmd3/1

== system rzs10thnew2021b/Motor_Control/Manual_Torque_Calculation ==
  sensor_signal : Inport
  Enable : EnablePort
  Add : Sum
  Bus Selector : BusSelector  OutputSignals=apps1,apps2
  Constant : Constant  Value=2
  Constant1 : Constant  Value=0
  Divide : Product  Inputs=*/
  Logical Operator : Logic  Operator=NOT  AllPortsSameDT=off  OutDataTypeStr=boolean
  Pedal_Fault_Check : Stateflow chart  TreatAsAtomicUnit=on
  Product : Product
  Switch : Switch  Criteria=u2 > Threshold
  max_torque : Constant  Value=50
  manual_torque : Outport
  wires:
  Bus Selector/1 -> Add/1, Pedal_Fault_Check/1(apps1)  "<apps1>"
  sensor_signal/1 -> Bus Selector/1
  Bus Selector/2 -> Pedal_Fault_Check/2(apps2), Add/2  "<apps2>"
  Add/1 -> Divide/1
  Constant/1 -> Divide/2
  Divide/1 -> Product/1
  max_torque/1 -> Product/2
  Switch/1 -> manual_torque/1
  Product/1 -> Switch/1
  Pedal_Fault_Check/1(pedal_error) -> Logical Operator/1
  Logical Operator/1 -> Switch/2
  Constant1/1 -> Switch/3

== system rzs10thnew2021b/Res/Res_Msg ==
  res_msg : Inport
  Bit Shift : hdlsllib/Logic and Bit Operations/Bit Shift  mode=Shift Right Logical  N=1
  Bit Shift1 : hdlsllib/Logic and Bit Operations/Bit Shift  mode=Shift Right Logical  N=2
  Bit Shift2 : hdlsllib/Logic and Bit Operations/Bit Shift  mode=Shift Right Logical  N=4
  Bitwise AND : simulink/Logic and Bit Operations/Bitwise Operator  logicop=AND  UseBitMask=on  BitMask=bin2dec('00000001')  BitMaskRealWorld=Stored Integer
  Bitwise AND1 : simulink/Logic and Bit Operations/Bitwise Operator  logicop=AND  UseBitMask=on  BitMask=bin2dec('00000010')  BitMaskRealWorld=Stored Integer
  Bitwise AND2 : simulink/Logic and Bit Operations/Bitwise Operator  logicop=AND  UseBitMask=on  BitMask=bin2dec('00000100')  BitMaskRealWorld=Stored Integer
  Bitwise AND3 : simulink/Logic and Bit Operations/Bitwise Operator  logicop=AND  UseBitMask=on  BitMask=bin2dec('00010000')  BitMaskRealWorld=Stored Integer
  Bitwise AND4 : simulink/Logic and Bit Operations/Bitwise Operator  logicop=AND  UseBitMask=on  BitMask=bin2dec('11111111')  BitMaskRealWorld=Stored Integer
  Bitwise AND5 : simulink/Logic and Bit Operations/Bitwise Operator  logicop=AND  UseBitMask=on  BitMask=bin2dec('11111111')  BitMaskRealWorld=Stored Integer
  Bus Creator : BusCreator  Inputs=5
  Data Type Conversion{1..3,7} (4 alike) : DataTypeConversion  OutDataTypeStr=boolean
  Demux : Demux  Outputs=8
  Logical Operator : Logic  Operator=XOR  AllPortsSameDT=off  OutDataTypeStr=boolean
  Subsystem : Subsystem
  Terminator{,1..4} (5 alike) : Terminator
  res_signal : Outport
  wires:
  res_msg/1 -> Demux/1
  Demux/1 -> Bitwise AND/1, Bitwise AND1/1, Bitwise AND3/1, Bitwise AND2/1, Logical Operator/1
  Bitwise AND/1 -> Data Type Conversion7/1
  Bitwise AND1/1 -> Bit Shift/1
  Bit Shift/1 -> Data Type Conversion1/1
  Bitwise AND2/1 -> Bit Shift1/1
  Data Type Conversion7/1 -> Bus Creator/1  "res_stop"
  Data Type Conversion1/1 -> Bus Creator/2  "res_gobutton"
  Bit Shift1/1 -> Data Type Conversion2/1
  Data Type Conversion2/1 -> Subsystem/1(res_communication), Bus Creator/3  "res_communication"
  Bitwise AND3/1 -> Bit Shift2/1
  Bit Shift2/1 -> Data Type Conversion3/1
  Data Type Conversion3/1 -> Bus Creator/4  "res_go"
  Demux/2 -> Logical Operator/2, Bitwise AND4/1
  Bitwise AND4/1 -> Subsystem/2(res_heartbeat)  "res_heartbeat"
  Demux/3 -> Bitwise AND5/1
  Bitwise AND5/1 -> Subsystem/3(res_xorcheck)  "res_xorcheck"
  Demux/5 -> Terminator/1
  Demux/4 -> Terminator1/1
  Demux/6 -> Terminator2/1
  Demux/7 -> Terminator3/1
  Demux/8 -> Terminator4/1
  Bus Creator/1 -> res_signal/1
  Subsystem/1(res_check) -> Bus Creator/5  "res_check"
  Logical Operator/1 -> Subsystem/4(xor_consequence)  "xor_consequence"

== system rzs10thnew2021b/Sensor_Signal/Subsystem ==
  note: % u为频率，r为车轮滚动半径y=u*36.0*pi/180.0*0.225*3.6
  f_frequency : Inport
  h_frequency : Inport  Port=2
  Constant : Constant  Value=180
  Constant1 : Constant  Value=0.225
  Constant2 : Constant  Value=3.6
  Constant3 : Constant  Value=180
  Divide : Product  Inputs=*/
  Divide1 : Product  Inputs=*/
  Gain : Gain  Gain=36
  Gain1 : Gain  Gain=3.1415
  Gain2 : Gain  Gain=36
  Gain3 : Gain  Gain=3.1415
  Product : Product
  Product1 : Product
  Product2 : Product
  wheel_speed_f : Outport
  wheel_speed_h : Outport  Port=2
  wires:
  f_frequency/1 -> Gain/1
  Gain/1 -> Gain1/1
  Gain1/1 -> Divide/1
  Constant1/1 -> Product/1
  Constant2/1 -> Product/2
  Constant/1 -> Divide/2
  Divide/1 -> Product1/1
  Product/1 -> Product2/1, Product1/2
  Product1/1 -> wheel_speed_f/1
  h_frequency/1 -> Gain2/1
  Gain2/1 -> Gain3/1
  Constant3/1 -> Divide1/2
  Gain3/1 -> Divide1/1
  Product2/1 -> wheel_speed_h/1
  Divide1/1 -> Product2/2

== system rzs10thnew2021b/EPS/EPS_ReceiveMsg/EPS_Send_Msg1 ==
  canb_epssendmsg1 : Inport
  Add : Sum  Inputs=-++
  Add1 : Sum  Inputs=+-
  Bus Creator : BusCreator  Inputs=7
  Constant : Constant  Value=12.8  OutDataTypeStr=double
  Constant1 : Constant  Value=1024  OutDataTypeStr=double
  Data Type Conversion{1..3,9} (4 alike) : DataTypeConversion  OutDataTypeStr=double
  Demux : Demux  Outputs=8
  Gain1 : Gain  Gain=256
  canb_epssendmsg1signal : Outport
  wires:
  canb_epssendmsg1/1 -> Demux/1
  Bus Creator/1 -> canb_epssendmsg1signal/1
  Demux/1 -> Bus Creator/1  "eps_workmode"
  Demux/2 -> Data Type Conversion9/1
  Demux/3 -> Bus Creator/3  "eps_errorcode1"
  Demux/5 -> Data Type Conversion2/1
  Demux/4 -> Data Type Conversion1/1
  Data Type Conversion3/1 -> Bus Creator/4  "eps_realangle"
  Demux/6 -> Bus Creator/5  "eps_midddlefeedback"
  Demux/7 -> Bus Creator/6  "eps_errorcode2"
  Demux/8 -> Bus Creator/7  "eps_sned_xor"
  Data Type Conversion9/1 -> Add1/1
  Constant/1 -> Add1/2
  Add1/1 -> Bus Creator/2  "eps_torque"
  Data Type Conversion1/1 -> Gain1/1
  Constant1/1 -> Add/1
  Data Type Conversion2/1 -> Add/3
  Add/1 -> Data Type Conversion3/1
  Gain1/1 -> Add/2  "eps_realangle"

== system rzs10thnew2021b/EPS/EPS_ReceiveMsg/EPS_Send_Msg2 ==
  canb_epssendmsg2 : Inport
  Add1 : Sum  Inputs=-++
  Add2 : Sum
  Add5 : Sum  Inputs=-++
  Bit Shift1 : hdlsllib/Logic and Bit Operations/Bit Shift  mode=Shift Left Logical  N=8
  Bus Creator : BusCreator  Inputs=5
  Constant1 : Constant  Value=1024  OutDataTypeStr=uint16
  Constant2 : Constant  Value=1024  OutDataTypeStr=uint16
  Data Type Conversion1 : DataTypeConversion  OutDataTypeStr=double
  Data Type Conversion{5..6,8,10} (4 alike) : DataTypeConversion  OutDataTypeStr=uint8
  Data Type Conversion2 : DataTypeConversion  OutDataTypeStr=double
  Data Type Conversion3 : DataTypeConversion  OutDataTypeStr=uint16
  Data Type Conversion4 : DataTypeConversion  OutDataTypeStr=uint16
  Demux : Demux  Outputs=8
  Gain1 : Gain  Gain=256
  Gain2 : Gain  Gain=256
  canb_epssendmsg2signal : Outport
  wires:
  canb_epssendmsg2/1 -> Demux/1
  Bus Creator/1 -> canb_epssendmsg2signal/1
  Demux/1 -> Bus Creator/1  "eps_mode"
  Demux/8 -> Bus Creator/5  "eps_send_cound"
  Data Type Conversion2/1 -> Bus Creator/4  "actual_angle"
  Data Type Conversion6/1 -> Gain2/1
  Data Type Conversion5/1 -> Add1/3
  Constant1/1 -> Add1/1
  Demux/7 -> Data Type Conversion5/1
  Gain2/1 -> Add1/2
  Demux/6 -> Data Type Conversion6/1
  Add1/1 -> Data Type Conversion2/1
  Data Type Conversion1/1 -> Bus Creator/3  "received_angle"
  Data Type Conversion8/1 -> Gain1/1
  Data Type Conversion10/1 -> Add5/3
  Constant2/1 -> Add5/1
  Demux/5 -> Data Type Conversion10/1
  Gain1/1 -> Add5/2
  Demux/4 -> Data Type Conversion8/1
  Add5/1 -> Data Type Conversion1/1
  Demux/3 -> Data Type Conversion4/1
  Demux/2 -> Data Type Conversion3/1
  Add2/1 -> Bus Creator/2  "received_command_number"
  Bit Shift1/1 -> Add2/1
  Data Type Conversion3/1 -> Bit Shift1/1
  Data Type Conversion4/1 -> Add2/2

== system rzs10thnew2021b/EPS/EPS_TransmitMsg/Subsystem2 ==
  eps_wheel_angle : Inport
  Add1 : Sum
  Constant1 : Constant  Value=1024  OutDataTypeStr=double
  Data Type Conversion4 : DataTypeConversion  OutDataTypeStr=double
  Data Type Conversion5 : DataTypeConversion  OutDataTypeStr=uint16
  Gain1 : Gain  Gain=5
  ipc_cmdangle : Outport
  wires:
  Constant1/1 -> Add1/1
  Add1/1 -> Data Type Conversion5/1
  Data Type Conversion4/1 -> Gain1/1
  Gain1/1 -> Add1/2
  eps_wheel_angle/1 -> Data Type Conversion4/1
  Data Type Conversion5/1 -> ipc_cmdangle/1

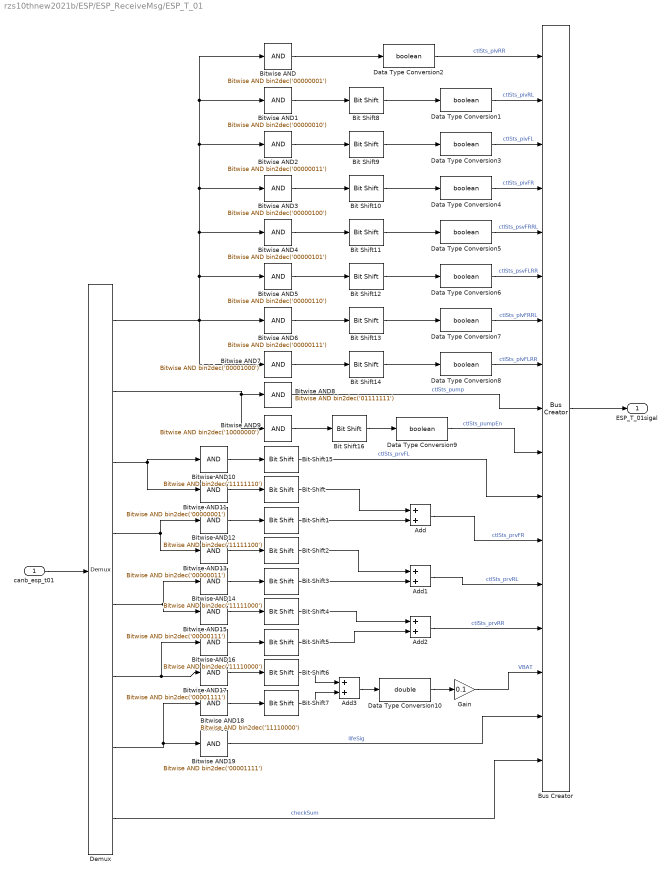
== system rzs10thnew2021b/ESP/ESP_ReceiveMsg/ESP_T_01 ==
  canb_esp_t01 : Inport
  Add{,1..3} (4 alike) : Sum
  Bit Shift : hdlsllib/Logic and Bit Operations/Bit Shift  mode=Shift Left Logical  N=6
  Bit Shift1 : hdlsllib/Logic and Bit Operations/Bit Shift  mode=Shift Right Logical  N=2
  Bit Shift10 : hdlsllib/Logic and Bit Operations/Bit Shift  mode=Shift Right Logical  N=3
  Bit Shift11 : hdlsllib/Logic and Bit Operations/Bit Shift  mode=Shift Right Logical  N=4
  Bit Shift12 : hdlsllib/Logic and Bit Operations/Bit Shift  mode=Shift Right Logical  N=5
  Bit Shift13 : hdlsllib/Logic and Bit Operations/Bit Shift  mode=Shift Right Logical  N=6
  Bit Shift14 : hdlsllib/Logic and Bit Operations/Bit Shift  mode=Shift Right Logical  N=7
  Bit Shift15 : hdlsllib/Logic and Bit Operations/Bit Shift  mode=Shift Right Logical  N=1
  Bit Shift16 : hdlsllib/Logic and Bit Operations/Bit Shift  mode=Shift Right Logical  N=7
  Bit Shift2 : hdlsllib/Logic and Bit Operations/Bit Shift  mode=Shift Left Logical  N=5
  Bit Shift3 : hdlsllib/Logic and Bit Operations/Bit Shift  mode=Shift Right Logical  N=3
  Bit Shift4 : hdlsllib/Logic and Bit Operations/Bit Shift  mode=Shift Left Logical  N=4
  Bit Shift5 : hdlsllib/Logic and Bit Operations/Bit Shift  mode=Shift Right Logical  N=4
  Bit Shift6 : hdlsllib/Logic and Bit Operations/Bit Shift  mode=Shift Left Logical  N=4
  Bit Shift7 : hdlsllib/Logic and Bit Operations/Bit Shift  mode=Shift Right Logical  N=4
  Bit Shift8 : hdlsllib/Logic and Bit Operations/Bit Shift  mode=Shift Right Logical  N=1
  Bit Shift9 : hdlsllib/Logic and Bit Operations/Bit Shift  mode=Shift Right Logical  N=2
  Bitwise AND : simulink/Logic and Bit Operations/Bitwise Operator  logicop=AND  UseBitMask=on  BitMask=bin2dec('00000001')  BitMaskRealWorld=Stored Integer
  Bitwise AND1 : simulink/Logic and Bit Operations/Bitwise Operator  logicop=AND  UseBitMask=on  BitMask=bin2dec('00000010')  BitMaskRealWorld=Stored Integer
  Bitwise AND10 : simulink/Logic and Bit Operations/Bitwise Operator  logicop=AND  UseBitMask=on  BitMask=bin2dec('11111110')  BitMaskRealWorld=Stored Integer
  Bitwise AND11 : simulink/Logic and Bit Operations/Bitwise Operator  logicop=AND  UseBitMask=on  BitMask=bin2dec('00000001')  BitMaskRealWorld=Stored Integer
  Bitwise AND12 : simulink/Logic and Bit Operations/Bitwise Operator  logicop=AND  UseBitMask=on  BitMask=bin2dec('11111100')  BitMaskRealWorld=Stored Integer
  Bitwise AND13 : simulink/Logic and Bit Operations/Bitwise Operator  logicop=AND  UseBitMask=on  BitMask=bin2dec('00000011')  BitMaskRealWorld=Stored Integer
  Bitwise AND14 : simulink/Logic and Bit Operations/Bitwise Operator  logicop=AND  UseBitMask=on  BitMask=bin2dec('11111000')  BitMaskRealWorld=Stored Integer
  Bitwise AND15 : simulink/Logic and Bit Operations/Bitwise Operator  logicop=AND  UseBitMask=on  BitMask=bin2dec('00000111')  BitMaskRealWorld=Stored Integer
  Bitwise AND16 : simulink/Logic and Bit Operations/Bitwise Operator  logicop=AND  UseBitMask=on  BitMask=bin2dec('11110000')  BitMaskRealWorld=Stored Integer
  Bitwise AND17 : simulink/Logic and Bit Operations/Bitwise Operator  logicop=AND  UseBitMask=on  BitMask=bin2dec('00001111')  BitMaskRealWorld=Stored Integer
  Bitwise AND18 : simulink/Logic and Bit Operations/Bitwise Operator  logicop=AND  UseBitMask=on  BitMask=bin2dec('11110000')  BitMaskRealWorld=Stored Integer
  Bitwise AND19 : simulink/Logic and Bit Operations/Bitwise Operator  logicop=AND  UseBitMask=on  BitMask=bin2dec('00001111')  BitMaskRealWorld=Stored Integer
  Bitwise AND2 : simulink/Logic and Bit Operations/Bitwise Operator  logicop=AND  UseBitMask=on  BitMask=bin2dec('00000011')  BitMaskRealWorld=Stored Integer
  Bitwise AND3 : simulink/Logic and Bit Operations/Bitwise Operator  logicop=AND  UseBitMask=on  BitMask=bin2dec('00000100')  BitMaskRealWorld=Stored Integer
  Bitwise AND4 : simulink/Logic and Bit Operations/Bitwise Operator  logicop=AND  UseBitMask=on  BitMask=bin2dec('00000101')  BitMaskRealWorld=Stored Integer
  Bitwise AND5 : simulink/Logic and Bit Operations/Bitwise Operator  logicop=AND  UseBitMask=on  BitMask=bin2dec('00000110')  BitMaskRealWorld=Stored Integer
  Bitwise AND6 : simulink/Logic and Bit Operations/Bitwise Operator  logicop=AND  UseBitMask=on  BitMask=bin2dec('00000111')  BitMaskRealWorld=Stored Integer
  Bitwise AND7 : simulink/Logic and Bit Operations/Bitwise Operator  logicop=AND  UseBitMask=on  BitMask=bin2dec('00001000')  BitMaskRealWorld=Stored Integer
  Bitwise AND8 : simulink/Logic and Bit Operations/Bitwise Operator  logicop=AND  UseBitMask=on  BitMask=bin2dec('01111111')  BitMaskRealWorld=Stored Integer
  Bitwise AND9 : simulink/Logic and Bit Operations/Bitwise Operator  logicop=AND  UseBitMask=on  BitMask=bin2dec('10000000')  BitMaskRealWorld=Stored Integer
  Bus Creator : BusCreator  Inputs=17
  Data Type Conversion{1..9} (9 alike) : DataTypeConversion  OutDataTypeStr=boolean
  Data Type Conversion10 : DataTypeConversion  OutDataTypeStr=double
  Demux : Demux  Outputs=8
  Gain : Gain  Gain=0.1
  ESP_T_01sigal : Outport
  wires:
  canb_esp_t01/1 -> Demux/1
  Bus Creator/1 -> ESP_T_01sigal/1
  Bitwise AND/1 -> Data Type Conversion2/1
  Demux/1 -> Bitwise AND/1, Bitwise AND1/1, Bitwise AND2/1, Bitwise AND3/1, Bitwise AND4/1, Bitwise AND5/1, Bitwise AND7/1, Bitwise AND6/1
  Demux/2 -> Bitwise AND9/1, Bitwise AND8/1
  Bitwise AND8/1 -> Bus Creator/9  "ctlSts_pump"
  Bitwise AND10/1 -> Bit Shift15/1
  Demux/4 -> Bitwise AND12/1, Bitwise AND13/1
  Demux/3 -> Bitwise AND10/1, Bitwise AND11/1
  Bitwise AND11/1 -> Bit Shift/1
  Bitwise AND12/1 -> Bit Shift1/1
  Bit Shift1/1 -> Add/2
  Bit Shift/1 -> Add/1
  Add/1 -> Bus Creator/12  "ctlSts_prvFR"
  Bitwise AND13/1 -> Bit Shift2/1
  Demux/5 -> Bitwise AND14/1, Bitwise AND15/1
  Bitwise AND14/1 -> Bit Shift3/1
  Bit Shift2/1 -> Add1/1
  Bit Shift3/1 -> Add1/2
  Add1/1 -> Bus Creator/13  "ctlSts_prvRL"
  Bitwise AND15/1 -> Bit Shift4/1
  Demux/6 -> Bitwise AND16/1, Bitwise AND17/1
  Bitwise AND16/1 -> Bit Shift5/1
  Bit Shift4/1 -> Add2/1
  Bit Shift5/1 -> Add2/2
  Add2/1 -> Bus Creator/14  "ctlSts_prvRR"
  Bitwise AND17/1 -> Bit Shift6/1
  Demux/7 -> Bitwise AND18/1, Bitwise AND19/1
  Bitwise AND18/1 -> Bit Shift7/1
  Bit Shift6/1 -> Add3/1
  Bit Shift7/1 -> Add3/2
  Bitwise AND19/1 -> Bus Creator/16  "lifeSig"
  Demux/8 -> Bus Creator/17  "checkSum"
  Bitwise AND1/1 -> Bit Shift8/1
  Bit Shift8/1 -> Data Type Conversion1/1
  Bitwise AND2/1 -> Bit Shift9/1
  Bit Shift9/1 -> Data Type Conversion3/1
  Bitwise AND3/1 -> Bit Shift10/1
  Bitwise AND4/1 -> Bit Shift11/1
  Bitwise AND5/1 -> Bit Shift12/1
  Bitwise AND6/1 -> Bit Shift13/1
  Bitwise AND7/1 -> Bit Shift14/1
  Bit Shift10/1 -> Data Type Conversion4/1
  Bit Shift11/1 -> Data Type Conversion5/1
  Bit Shift12/1 -> Data Type Conversion6/1
  Bit Shift13/1 -> Data Type Conversion7/1
  Bit Shift14/1 -> Data Type Conversion8/1
  Gain/1 -> Bus Creator/15  "VBAT"
  Data Type Conversion2/1 -> Bus Creator/1  "ctlSts_pivRR"
  Data Type Conversion1/1 -> Bus Creator/2  "ctlSts_pivRL"
  Data Type Conversion3/1 -> Bus Creator/3  "ctlSts_pivFL"
  Data Type Conversion4/1 -> Bus Creator/4  "ctlSts_pivFR"
  Data Type Conversion5/1 -> Bus Creator/5  "ctlSts_psvFRRL"
  Data Type Conversion6/1 -> Bus Creator/6  "ctlSts_psvFLRR"
  Data Type Conversion7/1 -> Bus Creator/7  "ctlSts_plvFRRL"
  Data Type Conversion8/1 -> Bus Creator/8  "ctlSts_plvFLRR"
  Bit Shift15/1 -> Bus Creator/11  "ctlSts_prvFL"
  Bitwise AND9/1 -> Bit Shift16/1
  Bit Shift16/1 -> Data Type Conversion9/1
  Data Type Conversion9/1 -> Bus Creator/10  "ctlSts_pumpEn"
  Data Type Conversion10/1 -> Gain/1
  Add3/1 -> Data Type Conversion10/1
